simulink model "fir"  (R2017b)
settings: Solver=FixedStepDiscrete  StartTime=0.0  StopTime=tstop  FixedStep=ts  RelTol=1e-3
values from neighbouring files (symbols this model uses):
  B0 = randn(p,q)    [runme.m]
  B1 = randn(p,q)    [runme.m]
  B2 = randn(p,q)    [runme.m]
  q = 3    [runme.m]
  ts = 1/100    (= 0.01)    [runme.m]
libraries: simulink x1
settings Model: Creator=jtesch  LastModifiedBy=jtesch

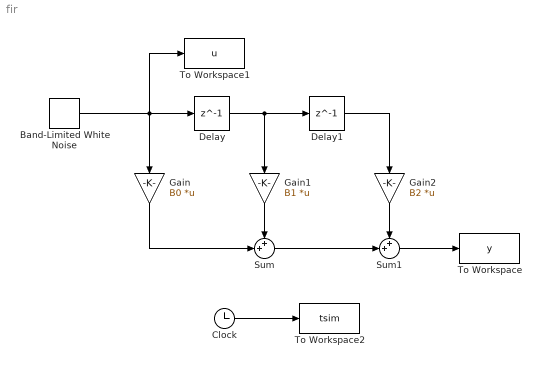
== system fir ==
  Band-Limited White Noise : simulink/Sources/Band-Limited White Noise  Cov=0.1*ones(q,1)  Ts=ts  seed=[23341]  VectorParams1D=off
  Clock : Clock
  Delay : Delay  DelayLength=1
  Delay1 : Delay  DelayLength=1
  Gain : Gain  Gain=B0  Multiplication=Matrix(K*u) (u vector)
  Gain1 : Gain  Gain=B1  Multiplication=Matrix(K*u) (u vector)
  Gain2 : Gain  Gain=B2  Multiplication=Matrix(K*u) (u vector)
  Sum : Sum  Inputs=++|
  Sum1 : Sum  Inputs=++|
  To Workspace : ToWorkspace  VariableName=y  SampleTime=-1
  To Workspace1 : ToWorkspace  VariableName=u  SampleTime=-1
  To Workspace2 : ToWorkspace  VariableName=tsim  SampleTime=-1
  wires:
  Band-Limited White Noise/1 -> To Workspace1/1, Gain/1, Delay/1
  Delay/1 -> Gain1/1, Delay1/1
  Delay1/1 -> Gain2/1
  Gain1/1 -> Sum/1
  Gain/1 -> Sum/2
  Sum/1 -> Sum1/2
  Gain2/1 -> Sum1/1
  Sum1/1 -> To Workspace/1
  Clock/1 -> To Workspace2/1
